simulink model "C172S_PitchRateDamper_V1"  (R2026a)
settings: Solver=ode4  StartTime=0  StopTime=12  FixedStep=0.01
InitFcn:
  | qdData = c172sLongitudinalData();
  | [~, qdPlant] = c172sLongitudinalPlant(qdData);
  | qdDamper = c172sPitchRateDamperData();
  | A_qd = qdPlant.A; B_qd = qdPlant.B;
  | C_qd = qdPlant.C; D_qd = qdPlant.D;
  | Kq_pitchRate_s = qdDamper.Kq_s;
  | qd_deltaECommand_rad = 0.0;
  | x0_qd = [0; 0; deg2rad(5.0); 0];
settings Model: Creator=Shahi  LastModifiedBy=Shahi

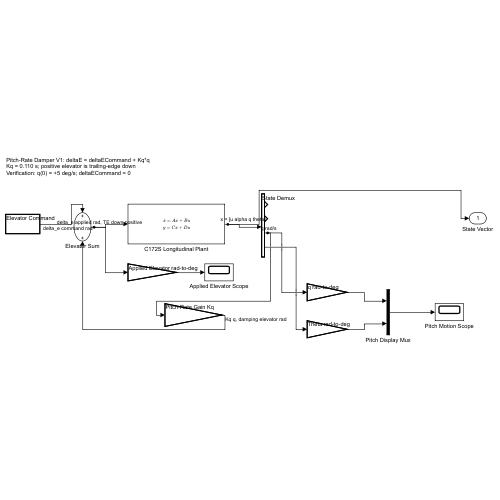
[thumbnail: Simulink's stored preview of the top-level diagram]
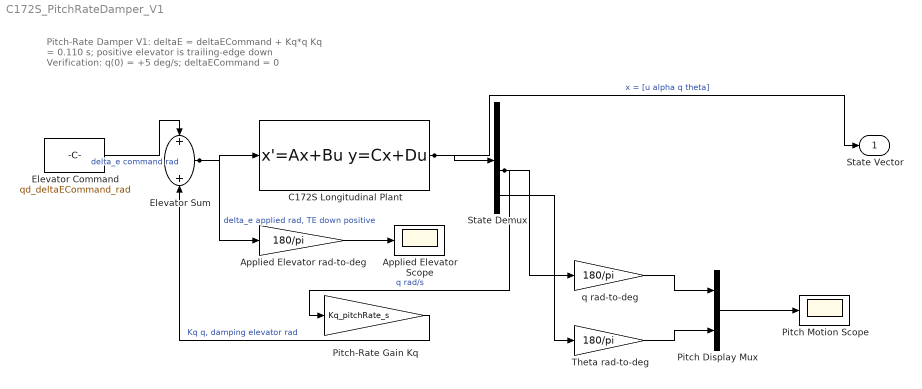
== system C172S_PitchRateDamper_V1 ==
  note: Pitch-Rate Damper V1: deltaE = deltaECommand + Kq*q
      | Kq = 0.110 s; positive elevator is trailing-edge down
      | Verification: q(0) = +5 deg/s; deltaECommand = 0
  Applied Elevator Scope : Scope
  Applied Elevator rad-to-deg : Gain  Gain=180/pi
  C172S Longitudinal Plant : StateSpace  A=A_qd  B=B_qd  C=C_qd  D=D_qd  InitialCondition=x0_qd
  Elevator Command : Constant  Value=qd_deltaECommand_rad  SampleTime=0
  Elevator Sum : Sum
  Pitch Display Mux : Mux  Inputs=2
  Pitch Motion Scope : Scope
  Pitch-Rate Gain Kq : Gain  Gain=Kq_pitchRate_s
  State Demux : Demux
  Theta rad-to-deg : Gain  Gain=180/pi
  q rad-to-deg : Gain  Gain=180/pi
  State Vector : Outport
  wires:
  Elevator Command/1 -> Elevator Sum/1  "delta_e command rad"
  Elevator Sum/1 -> C172S Longitudinal Plant/1, Applied Elevator rad-to-deg/1  "delta_e applied rad, TE down positive"
  Applied Elevator rad-to-deg/1 -> Applied Elevator Scope/1
  C172S Longitudinal Plant/1 -> State Vector/1, State Demux/1  "x = [u alpha q theta]"
  State Demux/3 -> Pitch-Rate Gain Kq/1, q rad-to-deg/1  "q rad/s"
  Pitch-Rate Gain Kq/1 -> Elevator Sum/2  "Kq q, damping elevator rad"
  q rad-to-deg/1 -> Pitch Display Mux/1
  State Demux/4 -> Theta rad-to-deg/1
  Theta rad-to-deg/1 -> Pitch Display Mux/2
  Pitch Display Mux/1 -> Pitch Motion Scope/1
